simulink model "my_library"  (R2016a)
settings: Solver=VariableStepAuto  StartTime=0.0  StopTime=2  MaxStep=0.01  RelTol=1e-4
libraries: simulink x1
settings Model: Creator=Administrator  LastModifiedBy=Administrator
settings DataIOCC: LimitDataPoints=on  SaveOutput=off  SaveTime=off
settings OptimizationCC: ExpressionDepthLimit=2147483647  LifeSpan=1
settings DebuggingCC: FcnCallInpInsideContextMsg=EnableAllAsWarning  AllowSymbolicDim=off  StateNameClashWarn=warning
settings GRTTargetCC: CombineOutputUpdateFcns=off  GRTInterface=on

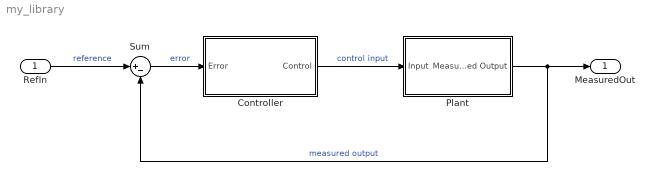
== system my_library ==
  RefIn : Inport
  Controller : Subsystem
  Plant : Subsystem
  Sum : Sum  Inputs=|+-
  MeasuredOut : Outport
  wires:
  RefIn/1 -> Sum/1  "reference"
  Plant/1(Measured Output) -> Sum/2, MeasuredOut/1  "measured output"
  Sum/1 -> Controller/1(Error)  "error"
  Controller/1(Control) -> Plant/1(Input)  "control input"

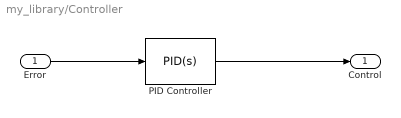
== system my_library/Controller ==
  Error : Inport
  PID Controller : simulink/Continuous/PID Controller  Controller=PID  TimeDomain=Continuous-time  SampleTime=-1  IntegratorMethod=Forward Euler  FilterMethod=Forward Euler  Form=Parallel  UseFilter=on  ControllerParametersSource=internal  P=1.2  I=22  D=0.02  N=20  InitialConditionSource=internal  InitialConditionForIntegrator=0  InitialConditionForFilter=0  ExternalReset=none  LimitOutput=off  UpperSaturationLimit=inf  LowerSaturationLimit=-inf  LinearizeAsGain=on  AntiWindupMode=none  Kb=1  TrackingMode=off  Kt=1  PParamMin=[]  PParamMax=[]  IParamMin=[]  IParamMax=[]  DParamMin=[]  DParamMax=[]  NParamMin=[]  NParamMax=[]  KbParamMin=[]  KbParamMax=[]  KtParamMin=[]  KtParamMax=[]  POutMin=[]  POutMax=[]  IOutMin=[]  IOutMax=[]  DOutMin=[]  DOutMax=[]  NOutMin=[]  NOutMax=[]  KbOutMin=[]  KbOutMax=[]  KtOutMin=[]  KtOutMax=[]  IntegratorOutMin=[]  IntegratorOutMax=[]  FilterOutMin=[]  FilterOutMax=[]  SumOutMin=[]  SumOutMax=[]  SumI1OutMin=[]  SumI1OutMax=[]  SumI2OutMin=[]  SumI2OutMax=[]  SumI3OutMin=[]  SumI3OutMax=[]  SumDOutMin=[]  SumDOutMax=[]  SaturationOutMin=[]  SaturationOutMax=[]  IntegratorContinuousStateAttributes=''  IntegratorStateMustResolveToSignalObject=off  IntegratorRTWStateStorageClass=Auto  FilterContinuousStateAttributes=''  FilterStateMustResolveToSignalObject=off  FilterRTWStateStorageClass=Auto  DifferentiatorICPrevScaledInput=0  DifferentiatorOutMin=[]  DifferentiatorOutMax=[]
  Control : Outport
  wires:
  Error/1 -> PID Controller/1
  PID Controller/1 -> Control/1

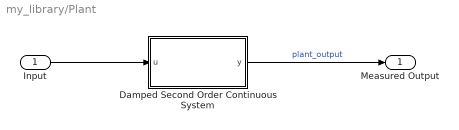
== system my_library/Plant ==
  Input : Inport
  Damped Second Order Continuous System : Subsystem  mask{wn=16, zeta=0.6}
      mask prompts: wn "Undamped natural frequency (wn, rad/s)"; zeta "Damping factor (zeta)"
  Measured Output : Outport
  wires:
  Input/1 -> Damped Second Order Continuous System/1(u)
  Damped Second Order Continuous System/1(y) -> Measured Output/1  "plant_output"

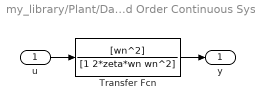
== system my_library/Plant/Damped Second Order Continuous System ==
  u : Inport
  Transfer Fcn : TransferFcn  Numerator=[wn^2]  Denominator=[1 2*zeta*wn wn^2]
  y : Outport
  wires:
  Transfer Fcn/1 -> y/1
  u/1 -> Transfer Fcn/1
